simulink model "Modele_non_lineaire_bis"  (R2023b)
settings: Solver=VariableStepAuto  StartTime=0.0  StopTime=100  MaxStep=1e-4  RelTol=1e-3
values from neighbouring files (symbols this model uses):
  delta0 = n_g / K_s * Tg0    [EI.m]
undefined symbols (not defined in the file or in its folder): x
settings Model: Creator=33783  LastModifiedBy=33783

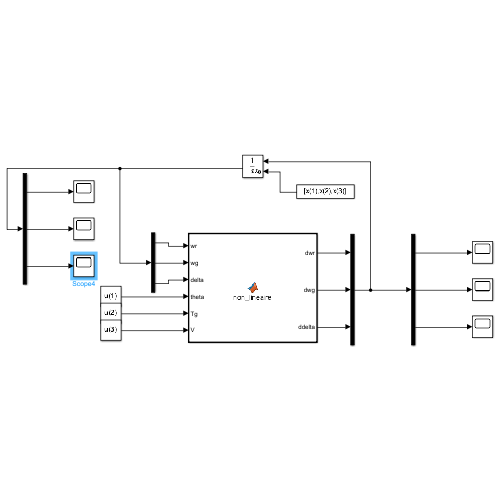
[thumbnail: Simulink's stored preview of the top-level diagram]
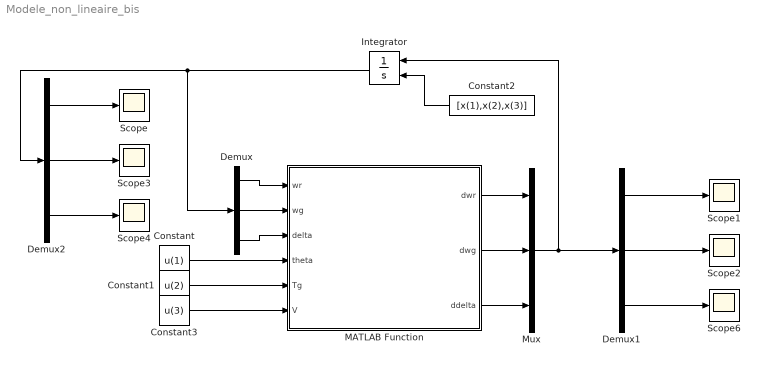
== system Modele_non_lineaire_bis ==
  Constant : Constant  Value=u(1)
  Constant1 : Constant  Value=u(2)
  Constant2 : Constant  Value=[x(1),x(2),x(3)]  VectorParams1D=off
  Constant3 : Constant  Value=u(3)
  Demux : Demux  Outputs=3
  Demux1 : Demux  Outputs=3
  Demux2 : Demux  Outputs=3
  Integrator : Integrator  InitialConditionSource=external  InitialCondition=[4.267,184.2,delta0]
  MATLAB Function : MATLAB Function  TreatAsAtomicUnit=on
  Mux : Mux  Inputs=3
  Scope{,1..4,6} (6 alike) : Scope
  wires:
  Mux/1 -> Integrator/1, Demux1/1
  MATLAB Function/1(dwr) -> Mux/1
  MATLAB Function/2(dwg) -> Mux/2
  Demux/1 -> MATLAB Function/1(wr)
  Demux/2 -> MATLAB Function/2(wg)
  Demux/3 -> MATLAB Function/3(delta)
  MATLAB Function/3(ddelta) -> Mux/3
  Integrator/1 -> Demux/1, Demux2/1
  Demux1/1 -> Scope1/1
  Demux1/3 -> Scope6/1
  Demux1/2 -> Scope2/1
  Constant2/1 -> Integrator/2
  Constant/1 -> MATLAB Function/4(theta)
  Constant1/1 -> MATLAB Function/5(Tg)
  Constant3/1 -> MATLAB Function/6(V)
  Demux2/1 -> Scope/1
  Demux2/2 -> Scope3/1
  Demux2/3 -> Scope4/1

== matlab function Modele_non_lineaire_bis/MATLAB Function ==
  data: wr input; dwr output; wg input; delta input; theta input; Tg input; dwg output; ddelta output; V input
function [dwr,dwg,ddelta] = non_lineaire(wr,wg,delta,theta,Tg,V)
    % Valeurs du modèle :
    n_g = 43.165 ; % sans unité
    J_r = 3.25e5; % kg/m^2
    J_g = 34.4 ; % kg/m^2
    K_s = 269.1e3 ; % N.m/rad
    R = 21.65 ; % en mètres
    rho = 1.225 ; % en kg/m3
    D_s= 9500; % Nm/rad/s
    
    function Lambdai = funLambdai(lambda,theta)
        Lambdai = 1/(1/(lambda+0.08*theta)- 0.035/(theta^3 + 1)) ;
    end
    
    function Cp = funCp(lambda,theta) 
        Cp = 0.5*(116/funLambdai(lambda,theta)-0.4*theta-5)*exp(-21/funLambdai(lambda,theta)) + 0.0068*lambda ;
    end

    function Pr = funPuissance(wr,theta,V)
        Pr = 0.5*rho*pi*(R^2)*(V^3)*funCp(wr*R/V,theta);
    end
    
    dwr = 1/(J_r*wr) * funPuissance(wr,theta,V) - (D_s/J_r) *  + (wr*D_s/(J_r*n_g)) * wg - (K_s/J_r) * delta ;
    dwg = (D_s/(J_g * n_g)) * wr - (D_s/(J_g * n_g^2)) * wg + (K_s/(J_g * n_g)) * delta - (1/J_g) * Tg ;
    ddelta = wr - 1/n_g * wg;
end
